simulink model "TP3_1_3"  (R2018a)
settings: Solver=ode45  StartTime=0.0  StopTime=10.0  RelTol=1e-3
libraries: dsparch4 x6, commchan3 x1
settings Model: Creator=10RS6N  LastModifiedBy=10RS5
settings DataIOCC: SaveFormat=StructureWithTime  ReturnWorkspaceOutputs=on
settings OptimizationCC: LifeSpan=inf
settings DebuggingCC: SFExecutionAtInitializationDiag=none
settings HardwareCC: ProdBitPerSizeT=32  ProdBitPerPtrDiffT=32  ProdWordSize=32  ProdHWDeviceType=Specified
settings SFSimCC: SimUseLocalCustomCode=on
settings RTWCC: RTWUseLocalCustomCode=on
settings CodeAppCC: StateflowObjectComments=on

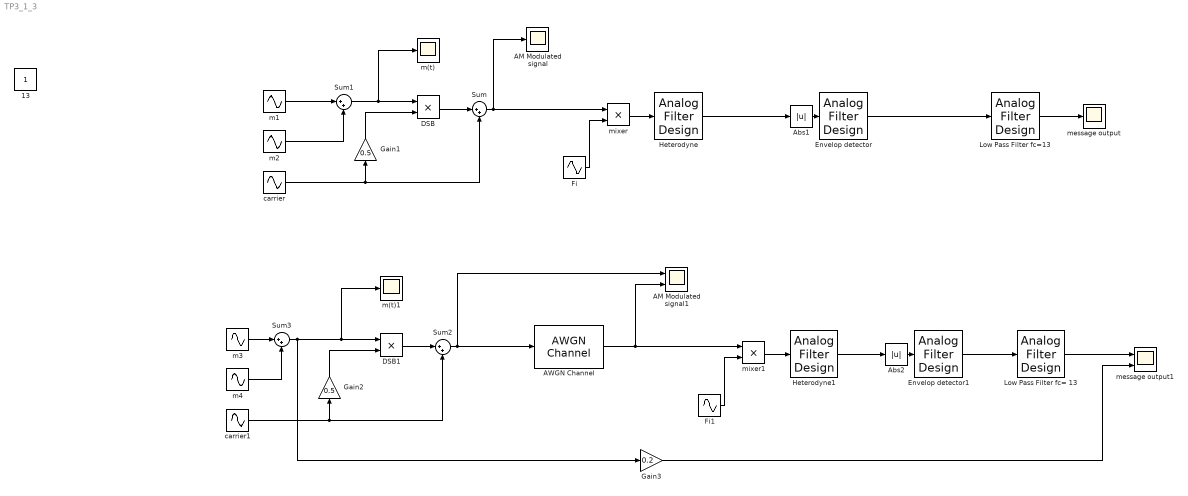
== system TP3_1_3 ==
  AM Modulated signal : Scope
  AM Modulated signal1 : Scope  NumInputPorts=2
  AWGN Channel : commchan3/AWGN Channel  InputProcessing=Columns as channels (frame based)  seed=67  noiseMode="Signal to noise ratio  (SNR)"  EbNodB=10  EsNodB=10  SNRdB=10  bitsPerSym=1  Ps=1  Tsym=1  variance=1
  Abs1 : Abs
  Abs2 : Abs
  DSB : Product
  DSB1 : Product
  Envelop detector : dsparch4/Analog Filter Design  method=Butterworth  filttype=Lowpass  N=6  Wlo=100*2*pi  Whi=1319.46  Rp=2  Rs=40
  Envelop detector1 : dsparch4/Analog Filter Design  method=Butterworth  filttype=Lowpass  N=6  Wlo=100*2*pi  Whi=1319.46  Rp=2  Rs=40
  Fi : Sin  Frequency=300*2*pi  SampleTime=0
  Fi1 : Sin  Frequency=300*2*pi  SampleTime=0
  Gain1 : Gain  Gain=0.5
  Gain2 : Gain  Gain=0.5
  Gain3 : Gain  Gain=0.2
  Heterodyne : dsparch4/Analog Filter Design  method=Butterworth  filttype=Bandpass  N=5  Wlo=187.8*2*pi  Whi=222*2*pi  Rp=2  Rs=40
  Heterodyne1 : dsparch4/Analog Filter Design  method=Butterworth  filttype=Bandpass  N=5  Wlo=187.8*2*pi  Whi=222*2*pi  Rp=2  Rs=40
  Low Pass Filter fc= 13 : dsparch4/Analog Filter Design  method=Butterworth  filttype=Lowpass  N=10  Wlo=13*2*pi  Whi=1319.46  Rp=2  Rs=40
  Low Pass Filter fc=13 : dsparch4/Analog Filter Design  method=Butterworth  filttype=Lowpass  N=10  Wlo=13*2*pi  Whi=1319.46  Rp=2  Rs=40
  Sum{,1..3} (4 alike) : Sum  Inputs=|++
  carrier : Sin  Frequency=500*2*pi  SampleTime=0
  carrier1 : Sin  Frequency=500*2*pi  SampleTime=0
  m(t) : Scope
  m(t)1 : Scope
  m1 : Sin  Frequency=5*2*pi  SampleTime=0
  m2 : Sin  Amplitude=0.5  Frequency=10*2*pi  SampleTime=0
  m3 : Sin  Frequency=5*2*pi  SampleTime=0
  m4 : Sin  Amplitude=0.5  Frequency=10*2*pi  SampleTime=0
  message output : Scope
  message output1 : Scope  NumInputPorts=2
  mixer : Product
  mixer1 : Product
  13 : Constant  IOType=siggen
  wires:
  m1/1 -> Sum1/1
  m2/1 -> Sum1/2
  Sum1/1 -> m(t)/1, DSB/1
  DSB/1 -> Sum/1
  carrier/1 -> Sum/2, Gain1/1
  Fi/1 -> mixer/2
  mixer/1 -> Heterodyne/1
  Heterodyne/1 -> Abs1/1
  Low Pass Filter fc=13/1 -> message output/1
  Gain1/1 -> DSB/2
  Sum/1 -> mixer/1, AM Modulated signal/1
  Abs1/1 -> Envelop detector/1
  Envelop detector/1 -> Low Pass Filter fc=13/1
  Envelop detector1/1 -> Low Pass Filter fc= 13/1
  Abs2/1 -> Envelop detector1/1
  Sum2/1 -> AM Modulated signal1/1, AWGN Channel/1
  Gain2/1 -> DSB1/2
  Low Pass Filter fc= 13/1 -> message output1/1
  Heterodyne1/1 -> Abs2/1
  mixer1/1 -> Heterodyne1/1
  Fi1/1 -> mixer1/2
  carrier1/1 -> Gain2/1, Sum2/2
  DSB1/1 -> Sum2/1
  m4/1 -> Sum3/2
  m3/1 -> Sum3/1
  AWGN Channel/1 -> AM Modulated signal1/2, mixer1/1
  Sum3/1 -> Gain3/1, DSB1/1, m(t)1/1
  Gain3/1 -> message output1/2
